simulink model "uavPackageDelivery"  (R2021b)
settings: Solver=VariableStepAuto  StartTime=0.0  StopTime=simTime  FixedStep=.005  RelTol=1e-3  EnableMultiTasking=on
undefined symbols (not defined in the file): baseMission, Earth, Newton, oaMission, Raphson, uavIC_latLon, UAVSampleTime, WGS84
libraries: aerolibtransform2 x1, robotalgslib x1
settings Model: DataDictionary=uavPackageDeliveryDataDict.sldd  ModifiedByFormat=The MathWorks, Inc.  Creator=The MathWorks, Inc.  LastModifiedBy=The MathWorks, Inc.
settings SolverCC: AlgebraicLoopSolver=TrustRegion  AutoInsertRateTranBlk=on
settings DataIOCC: LimitDataPoints=on  ReturnWorkspaceOutputs=off
settings OptimizationCC: DefaultParameterBehavior=Inlined  DefaultUnderspecifiedDataType=single  EnhancedBackFolding=on  PassReuseOutputArgsThreshold=0  MaxStackSize=64  OptimizeBlockOrder=speed  DifferentSizesBufferReuse=on  OptimizationCustomize=off
settings DebuggingCC: ParameterPrecisionLossMsg=none  ParameterTunabilityLossMsg=error  AllowSymbolicDim=off  SFUnexpectedBacktrackingDiag=warning  SFNoUnconditionalDefaultTransitionDiag=warning  SFExecutionAtInitializationDiag=none  SFMachineParentedDataDiag=warning  ArithmeticOperatorsInVariantConditions=warning
settings HardwareCC: ProdBitPerPointer=32  ProdBitPerSizeT=32  ProdBitPerPtrDiffT=32  ProdLargestAtomicFloat=None  ProdIntDivRoundTo=Undefined  ProdEndianess=Unspecified  ProdWordSize=32  ProdHWDeviceType=Generic->Unspecified (assume 32-bit Generic)
settings ModelReferenceCC: PropagateSignalLabelsOutOfModel=off
settings SFSimCC: SimUseLocalCustomCode=off  SimParseCustomCode=off  CustomCodeUndefinedFunction=UseInterfaceOnly
settings RTWCC: GenerateReport=on  RTWUseLocalCustomCode=off  LaunchReport=on
settings CodeAppCC: ForceParamTrailComments=on  OperatorAnnotations=on
settings GRTTargetCC: TargetLangStandard=C89/C90 (ANSI)
settings ConfigComp: CovMetricSettings=dw  CovSaveCumulativeToWorkspaceVar=on  CovSaveSingleToWorkspaceVar=on  CovExternalEMLEnable=off

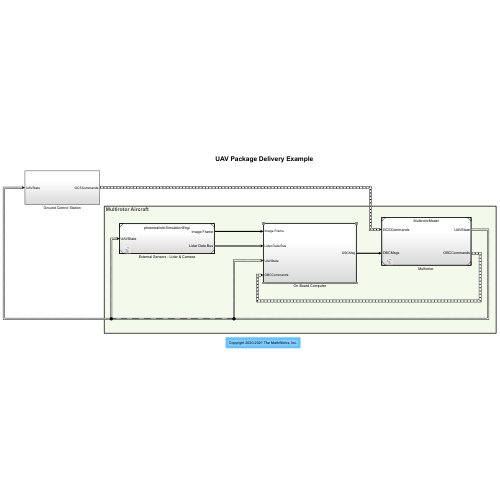
[thumbnail: Simulink's stored preview of the top-level diagram]
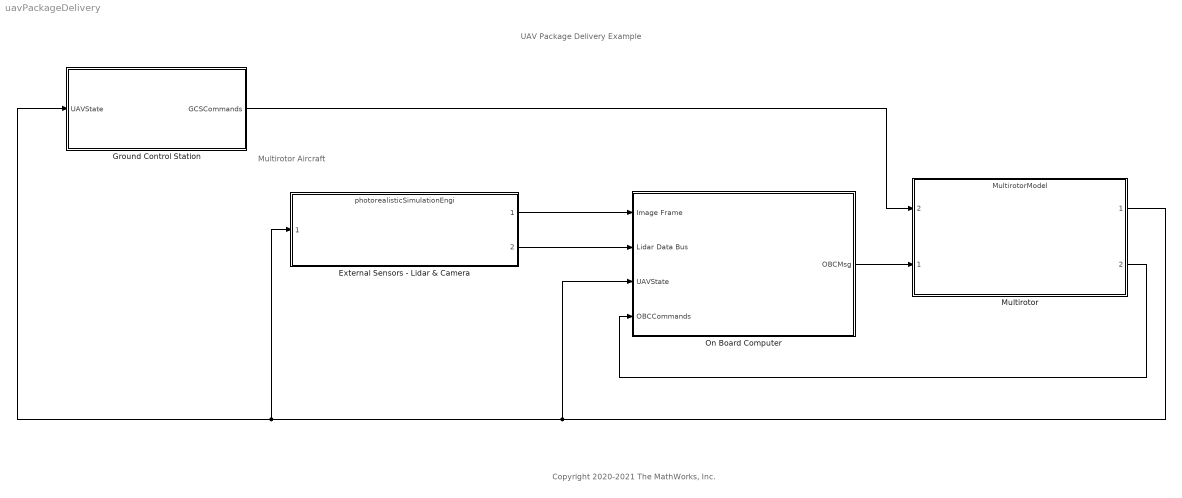
== system uavPackageDelivery ==
  note: Multirotor Aircraft
  note: UAV Package Delivery Example
  note: Copyright 2020-2021 The MathWorks, Inc.
  External Sensors - Lidar & Camera : ModelReference  ModelNameDialog=photorealisticSimulationEngi.slx  SimulationMode=Normal  ModelReferenceVersion=3.13
  Ground Control Station : Subsystem
  "Multirotor " : ModelReference  ModelNameDialog=MultirotorModel  SimulationMode=Normal  ModelReferenceVersion=4.68
      settings: PortSchema="{\"entries\":[{\"content\":{\"sides\":[{\"content\":{\"connectorIds\":[\"In2\",\"In1\"]},\"type\":\"ConnectorPlacement.EquallySpacedRectSide\",\"uuid\":\"abf53b88-b4c0-4cc3-bb4c-819ba68ade90\"},{\"content\":{\"connectorIds\":[\"Out1\",\"Out2\"],\"side\":\"RIGHT\"},\"type\":\"ConnectorPlacement.EquallySpacedRectSide\",\"uuid\":\"f1944fd3-3680-4558-bd6a-ffb0187ae725\"},{\"content\":{\"connectorIds\":[],\"side\":\"TOP\"},\"type\":\"ConnectorPlacement.EquallySpacedRectSide\",\"uuid\":\"7f686bac-a1b4-4e90-bc1f-e4dd6e8ae5c6\"}]},\"type\":\"ConnectorPlacement.EquallySpacedConnector\",\"uuid\":\"3f45c06a-90ee-44cf-add7-da13163a6845\"}],\"packageUris\":[\"http://schema.mathworks.com/mf0/Connector/R2020b\"],\"version\":\"1.0\"}"
  On Board Computer : Subsystem  TreatAsAtomicUnit=on
  wires:
  External Sensors - Lidar & Camera/1 -> On Board Computer/1(Image Frame)
  On Board Computer/1(OBCMsg) -> "Multirotor "/1
  External Sensors - Lidar & Camera/2 -> On Board Computer/2("Lidar Data Bus ")
  "Multirotor "/1 -> Ground Control Station/1(UAVState), External Sensors - Lidar & Camera/1, On Board Computer/3(UAVState)
  "Multirotor "/2 -> On Board Computer/4(OBCCommands)
  Ground Control Station/1(GCSCommands) -> "Multirotor "/2

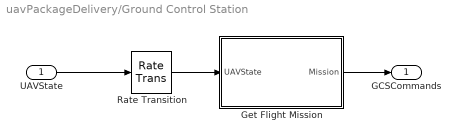
== system uavPackageDelivery/Ground Control Station ==
  UAVState : Inport  OutDataTypeStr=Bus: uavStateBus
  Get Flight Mission : Subsystem  Variant=on
  Rate Transition : RateTransition  OutPortSampleTime=UAVSampleTime*4
  GCSCommands : Outport
  wires:
  UAVState/1 -> Rate Transition/1
  Get Flight Mission/1("Mission ") -> GCSCommands/1
  Rate Transition/1 -> Get Flight Mission/1(UAVState)

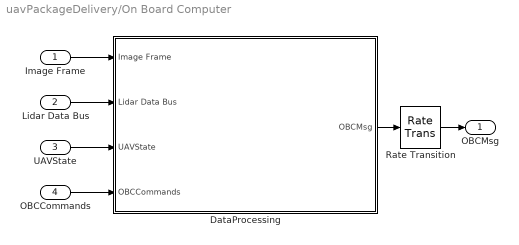
== system uavPackageDelivery/On Board Computer ==
  Image Frame : Inport
  "Lidar Data Bus " : Inport  Port=2
  UAVState : Inport  Port=3  OutDataTypeStr=Bus: uavStateBus  SampleTime=UAVSampleTime  BusOutputAsStruct=on
  OBCCommands : Inport  Port=4
  DataProcessing : Subsystem  Variant=on  PropagateVariantConditions=on
  Rate Transition : RateTransition  OutPortSampleTime=UAVSampleTime*4
  OBCMsg : Outport  OutDataTypeStr=single
  wires:
  Image Frame/1 -> DataProcessing/1(Image Frame)
  "Lidar Data Bus "/1 -> DataProcessing/2("Lidar Data Bus ")
  UAVState/1 -> DataProcessing/3(UAVState)
  OBCCommands/1 -> DataProcessing/4(OBCCommands)
  DataProcessing/1(OBCMsg) -> Rate Transition/1
  Rate Transition/1 -> OBCMsg/1

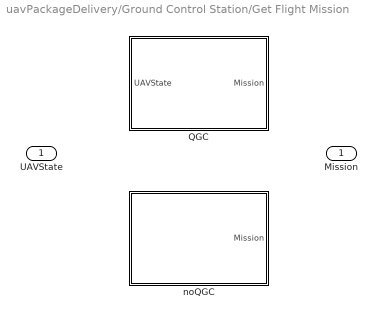
== system uavPackageDelivery/Ground Control Station/Get Flight Mission ==
  UAVState : Inport
  QGC : Subsystem  TreatAsAtomicUnit=on  SystemSampleTime=UAVSampleTime*4  VariantControl=useQGC==1
  noQGC : Subsystem  TreatAsAtomicUnit=on  SystemSampleTime=UAVSampleTime*4  VariantControl=useQGC==0
  "Mission " : Outport

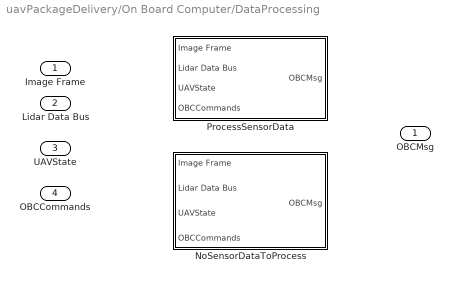
== system uavPackageDelivery/On Board Computer/DataProcessing ==
  Image Frame : Inport
  "Lidar Data Bus " : Inport  Port=2
  UAVState : Inport  Port=3  OutDataTypeStr=Bus: uavStateBus  SampleTime=0.005  BusOutputAsStruct=on
  OBCCommands : Inport  Port=4
  NoSensorDataToProcess : Subsystem  VariantControl=isPhotoRealisticSim==0
  ProcessSensorData : Subsystem  VariantControl=isPhotoRealisticSim ==1 || isPhotoRealisticSim ==2
  OBCMsg : Outport  OutDataTypeStr=single  SampleTime=0.005

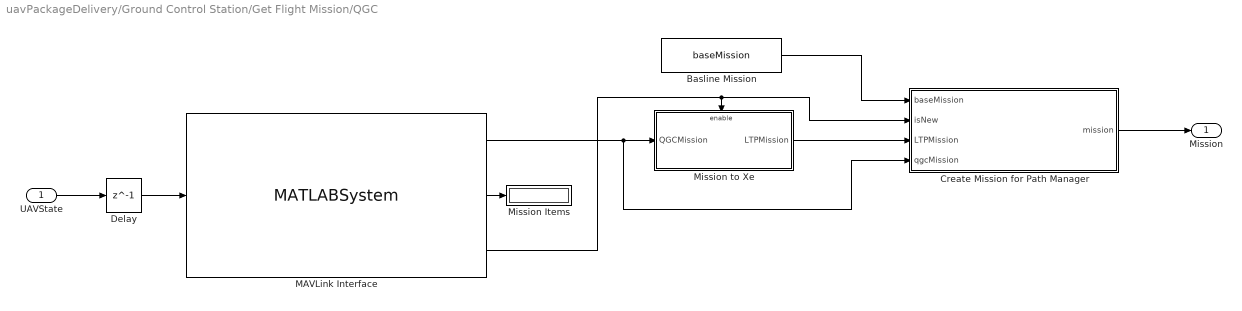
== system uavPackageDelivery/Ground Control Station/Get Flight Mission/QGC ==
  UAVState : Inport  OutDataTypeStr=Bus: uavStateBus
  Basline Mission : Constant  Value=baseMission  OutDataTypeStr=Bus: uavPathManagerBus  SampleTime=-1
  Create Mission for Path Manager : MATLAB Function  TreatAsAtomicUnit=on
  Delay : Delay  DelayLength=1
  MAVLink Interface : MATLABSystem  System=MAVLinkInterface  GCSPort=14550  MaxMissionLength=42  homeLatitude=uavIC_latLon(1)  homeLongitude=uavIC_latLon(2)
      mask Type: MAVLinkInterface
      mask Display:
      | disp('MAVLinkInterface');
      | port_label('input',1,'UAVState');
      | port_label('output',1,'missionItems');
      | port_label('output',2,'missionCount');
      | port_label('output',3,'uploadComplete');
  Mission Items : Display
  Mission to Xe : Subsystem
  Mission : Outport  OutDataTypeStr=Bus: uavPathManagerBus
  wires:
  MAVLink Interface/3 -> Create Mission for Path Manager/2(isNew), Mission to Xe/Enable
  Basline Mission/1 -> Create Mission for Path Manager/1(baseMission)
  Mission to Xe/1(LTPMission) -> Create Mission for Path Manager/3(LTPMission)
  Create Mission for Path Manager/1(mission) -> Mission/1
  MAVLink Interface/1 -> Mission to Xe/1(QGCMission), Create Mission for Path Manager/4(qgcMission)
  Delay/1 -> MAVLink Interface/1
  UAVState/1 -> Delay/1
  MAVLink Interface/2 -> Mission Items/1

== system uavPackageDelivery/Ground Control Station/Get Flight Mission/noQGC ==
  Variant Source : VariantSource
  Waypoints : Constant  Value=baseMission  OutDataTypeStr=Bus: uavPathManagerBus  SampleTime=-1
  Waypoints1 : Constant  Value=oaMission  OutDataTypeStr=Bus: uavPathManagerBus  SampleTime=-1
  Mission : Outport
  wires:
  Waypoints/1 -> Variant Source/1
  Waypoints1/1 -> Variant Source/2
  Variant Source/1 -> Mission/1

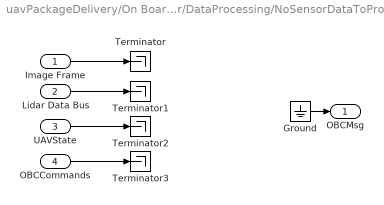
== system uavPackageDelivery/On Board Computer/DataProcessing/NoSensorDataToProcess ==
  Image Frame : Inport
  "Lidar Data Bus " : Inport  Port=2
  UAVState : Inport  Port=3  OutDataTypeStr=Bus: uavStateBus  SampleTime=UAVSampleTime  BusOutputAsStruct=on
  OBCCommands : Inport  Port=4
  Ground : Ground
  Terminator{,1..3} (4 alike) : Terminator
  OBCMsg : Outport  OutDataTypeStr=single  SampleTime=UAVSampleTime
  wires:
  Ground/1 -> OBCMsg/1
  Image Frame/1 -> Terminator/1
  "Lidar Data Bus "/1 -> Terminator1/1
  UAVState/1 -> Terminator2/1
  OBCCommands/1 -> Terminator3/1

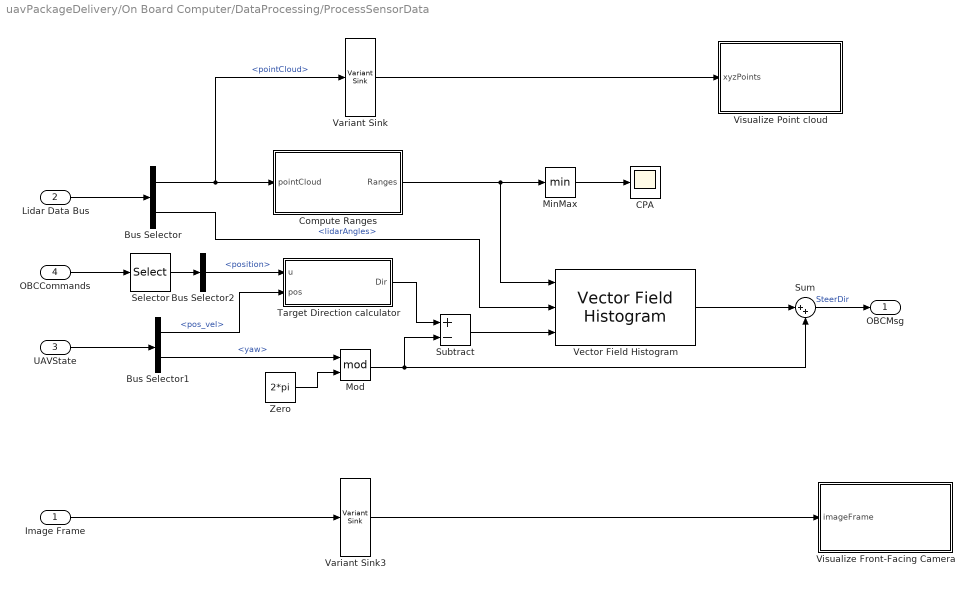
== system uavPackageDelivery/On Board Computer/DataProcessing/ProcessSensorData ==
  Image Frame : Inport
  "Lidar Data Bus " : Inport  Port=2  SampleTime=UAVSampleTime*10
  UAVState : Inport  Port=3  OutDataTypeStr=Bus: uavStateBus  SampleTime=UAVSampleTime*10  BusOutputAsStruct=on
  OBCCommands : Inport  Port=4  SampleTime=UAVSampleTime*10
  Bus Selector : BusSelector  OutputSignals=pointCloud,lidarAngles
  Bus Selector1 : BusSelector  OutputSignals=pos_vel,attitude.yaw
  Bus Selector2 : BusSelector  OutputSignals=position
  CPA : Scope
  Compute Ranges : Subsystem
  MinMax : MinMax
  Mod : Math  Operator=mod  SaturateOnIntegerOverflow=on
  Selector : Selector  InputPortWidth=2  IndexOptions=Index vector (dialog)  Indices=[2]  OutputSizes=1
  Subtract : Sum  Inputs=+-
  Sum : Sum  Inputs=|++  AccumDataTypeStr=single
  Target Direction calculator : MATLAB Function  TreatAsAtomicUnit=on
  Variant Sink : VariantSink
      settings: AllowZeroVariantControls=on
  Variant Sink3 : VariantSink
      settings: AllowZeroVariantControls=on
  Vector Field Histogram : robotalgslib/Vector Field Histogram  NumAngularSectors=360  DistanceLimits=[ 0 , 30 ]  HistogramThresholds=[ 5, 10 ]  RobotRadius=.5  SafetyDistance=0.65  MinTurningRadius=2  SimulateUsing=Code generation  TargetDirectionWeight=5  CurrentDirectionWeight=2  PreviousDirectionWeight=2
      settings: SourceProductBaseCode=NV,RO
  Visualize Front-Facing Camera : MATLAB Function  TreatAsAtomicUnit=on
  Visualize Point cloud : MATLAB Function  StopFcn=|  TreatAsAtomicUnit=on
      | playerFigure = findall(groot,'type','figure','name','Point Cloud Player');
      | 
      | if ~isempty(playerFigure)
      |     playerFigure = playerFigure(end);
      |     if isvalid(playerFigure)
      |         close(playerFigure);
      |     end
      | end
  Zero : Constant  Value=2*pi  OutDataTypeStr=Inherit: Inherit via back propagation
  OBCMsg : Outport  OutDataTypeStr=single  SampleTime=0.005
  wires:
  Bus Selector/1 -> Compute Ranges/1(pointCloud), Variant Sink/1  "<pointCloud>"
  Bus Selector1/1 -> Target Direction calculator/2(pos)  "<pos_vel>"
  Variant Sink/1 -> Visualize Point cloud/1(xyzPoints)
  Mod/1 -> Sum/2, Subtract/2
  MinMax/1 -> CPA/1
  Sum/1 -> OBCMsg/1  "SteerDir"
  Compute Ranges/1(Ranges) -> MinMax/1, Vector Field Histogram/1
  Vector Field Histogram/1 -> Sum/1
  Subtract/1 -> Vector Field Histogram/3
  OBCCommands/1 -> Selector/1
  Target Direction calculator/1(Dir) -> Subtract/1
  Variant Sink3/1 -> Visualize Front-Facing Camera/1(imageFrame)
  UAVState/1 -> Bus Selector1/1
  Bus Selector2/1 -> Target Direction calculator/1(u)  "<position>"
  Bus Selector/2 -> Vector Field Histogram/2  "<lidarAngles>"
  Zero/1 -> Mod/2
  Image Frame/1 -> Variant Sink3/1
  Selector/1 -> Bus Selector2/1
  Bus Selector1/2 -> Mod/1  "<yaw>"
  "Lidar Data Bus "/1 -> Bus Selector/1

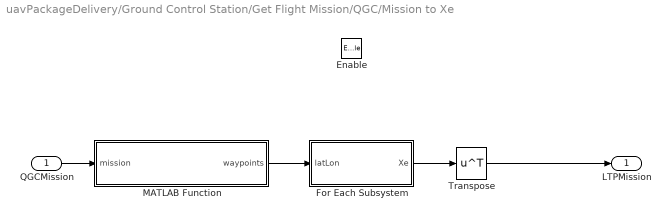
== system uavPackageDelivery/Ground Control Station/Get Flight Mission/QGC/Mission to Xe ==
  QGCMission : Inport
  Enable : EnablePort
  For Each Subsystem : Subsystem  TreatAsAtomicUnit=on
  MATLAB Function : MATLAB Function  TreatAsAtomicUnit=on
  Transpose : Math  Operator=transpose  SaturateOnIntegerOverflow=on
  LTPMission : Outport
  wires:
  For Each Subsystem/1(Xe) -> Transpose/1
  MATLAB Function/1(waypoints) -> For Each Subsystem/1(latLon)
  QGCMission/1 -> MATLAB Function/1(mission)
  Transpose/1 -> LTPMission/1

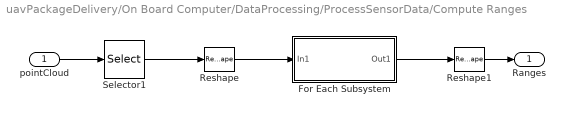
== system uavPackageDelivery/On Board Computer/DataProcessing/ProcessSensorData/Compute Ranges ==
  pointCloud : Inport
  For Each Subsystem : Subsystem  TreatAsAtomicUnit=on
  Reshape : Reshape  OutputDimensionality=Customize  OutputDimensions=[1083 3]
  Reshape1 : Reshape  OutputDimensions=1083
  Selector1 : Selector  NumberOfDimensions=3  InputPortWidth=3  IndexOptions=Index vector (dialog),Select all,Select all  Indices=16,1,1  OutputSizes=1,1,1
  Ranges : Outport
  wires:
  For Each Subsystem/1(Out1) -> Reshape1/1
  Selector1/1 -> Reshape/1
  pointCloud/1 -> Selector1/1
  Reshape/1 -> For Each Subsystem/1(In1)
  Reshape1/1 -> Ranges/1

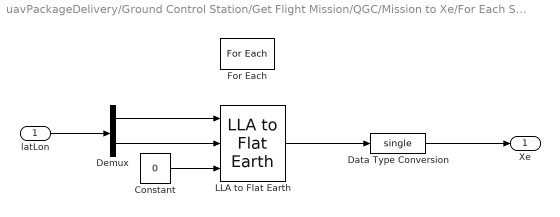
== system uavPackageDelivery/Ground Control Station/Get Flight Mission/QGC/Mission to Xe/For Each Subsystem ==
  latLon : Inport  Partition=on  PartitionDimension=1  PartitionWidth=1  PartitionOffset=0
  Constant : Constant  Value=0  OutDataTypeStr=double
  Data Type Conversion : DataTypeConversion  OutDataTypeStr=single
  Demux : Demux  Outputs=[2 1]
  For Each : ForEach  DisableCoverage=on
  LLA to Flat Earth : aerolibtransform2/LLA to Flat Earth  units=Metric (MKS)  ptype=Earth (WGS84)  F=1/298.257223563  R=6378137  refPosPort=off  LL0=uavIC_latLon  psi=0
      settings: SourceProductName=Aerospace Blockset
  Xe : Outport  ConcatenationDimension=2
  wires:
  LLA to Flat Earth/1 -> Data Type Conversion/1
  Demux/2 -> LLA to Flat Earth/2
  Demux/1 -> LLA to Flat Earth/1
  latLon/1 -> Demux/1
  Constant/1 -> LLA to Flat Earth/3
  Data Type Conversion/1 -> Xe/1

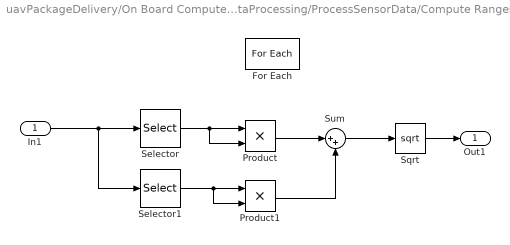
== system uavPackageDelivery/On Board Computer/DataProcessing/ProcessSensorData/Compute Ranges/For Each Subsystem ==
  In1 : Inport  Partition=on  PartitionDimension=1  PartitionWidth=1  PartitionOffset=0
  For Each : ForEach  DisableCoverage=on
  Product : Product
  Product1 : Product
  Selector : Selector  InputPortWidth=3  IndexOptions=Index vector (dialog)  Indices=[1]  OutputSizes=1
  Selector1 : Selector  InputPortWidth=3  IndexOptions=Index vector (dialog)  Indices=[2]  OutputSizes=1
  Sqrt : Sqrt  OutputSignalType=real  OutDataTypeStr=single  IntermediateResultsDataTypeStr=single  AlgorithmType=Newton-Raphson  SaturateOnIntegerOverflow=on
  Sum : Sum  Inputs=|++
  Out1 : Outport  ConcatenationDimension=1
  wires:
  In1/1 -> Selector1/1, Selector/1
  Selector/1 -> Product/2, Product/1
  Selector1/1 -> Product1/2, Product1/1
  Product/1 -> Sum/1
  Product1/1 -> Sum/2
  Sum/1 -> Sqrt/1
  Sqrt/1 -> Out1/1

== matlab function uavPackageDelivery/On Board Computer/DataProcessing/ProcessSensorData/Visualize Front-Facing Camera ==
  data: imageFrame input
function plotImageFrame(imageFrame)

coder.extrinsic('ishandle','image');

persistent fig;

if isempty(fig)
    fig = figure();
    ax = newplot(fig);
    title(ax, 'Front-facing camera');
end

if ~isempty(fig) && ishandle(fig)
    ax = newplot(fig);
    image(ax, imageFrame);
    axis(ax, 'off');
end

== matlab function uavPackageDelivery/Ground Control Station/Get Flight Mission/QGC/Mission to Xe/MATLAB Function ==
  data: mission input Bus: uavPathManagerBus size=42; waypoints output single size=[42 3]
function waypoints  = buildUAVMission(mission)
%
waypoints = single(zeros(42,3));

for i=1:length(mission)
    waypoints(i,1:3) = mission(i).position;
end

end

== matlab function uavPackageDelivery/Ground Control Station/Get Flight Mission/QGC/Create Mission for Path Manager ==
  data: baseMission input Bus: uavPathManagerBus size=42; isNew input size=1; LTPMission input size=[42 3]; mission output Bus: uavPathManagerBus size=42; qgcMission input Bus: uavPathManagerBus size=42
function mission = generateWaypointStream(baseMission, isNew, LTPMission, qgcMission)

persistent UAVMission

if isempty(UAVMission)
    UAVMission = baseMission;
end

%% If we got a new mission
if (isNew == true)
   for ii=1:42
       if LTPMission(ii,2) < 7275326
           UAVMission(ii).position = LTPMission(ii,:)';
           y = isnan(qgcMission(ii).params);
           UAVMission(ii).params = qgcMission(ii).params;
           if sum(y)>0
               UAVMission(ii).params(y) = single(0);
           end
           UAVMission(ii).mode = mavlinkToPlannerType(qgcMission(ii).mode);
       end
   end
end

mission = UAVMission;

end

function plannerType =  mavlinkToPlannerType (mavlinkType)
% see enum name="MAV_CMD" in common.xml for values.
    switch mavlinkType
        case 16 %MAV_CMD_NAV_WAYPOINT
            plannerType = uint8(2);
        case 18 %MAV_CMD_NAV_LOITER_TURNS
            plannerType = uint8(3);
        case 21 %MAV_CMD_NAV_LAND
            plannerType = uint8(4);
        case 22 %MAV_CMD_NAV_TAKEOFF
            plannerType = uint8(1);
        otherwise %this will likely error out to signal something unexpected
            plannerType = uint8(0);
    end
end

== matlab function uavPackageDelivery/On Board Computer/DataProcessing/ProcessSensorData/Target Direction calculator ==
  data: u input; Dir output; pos input
function Dir = TargetDir(u, pos)

Dir = atan2(u(2)-pos.y, u(1)-pos.x);

end

== matlab function uavPackageDelivery/On Board Computer/DataProcessing/ProcessSensorData/Visualize Point cloud ==
  data: xyzPoints input
function VisualizePointCloud(xyzPoints)
%VisualizePointCloud Display point cloud

coder.extrinsic('isOpen', 'pcplayer')

persistent player;

if isempty(player)
    % Configure axes limits
    xlimits = [-90 90];
    ylimits = [-90 90];
    zlimits = [ -50 50];
    
    % Create a streaming Lidar viewer
    player = pcplayer(xlimits, ylimits, zlimits);
end

if ~isempty(player) && isOpen(player)
    view(player, xyzPoints);
end
